simulink model "IM2_IndirectVector"  (R2022a)
settings: Solver=ode45  StartTime=0.0  StopTime=2  MaxStep=1e-5  RelTol=1e-3
values from neighbouring files (symbols this model uses):
  Vdc = 300    [IM2_Vector.m]    (also in Induction_motor_parameter.m)
undefined symbols (not defined in the file or in its folder): DCMotor, DiscIntNeverNeededParam, IM, INV1, INV2
libraries: simulink x3
settings Model: Creator=jun  LastModifiedBy=jun
settings DebuggingCC: UnconnectedInputMsg=warning  UnconnectedOutputMsg=warning  UnconnectedLineMsg=warning
settings RTWCC: DLArmComputeVersion=19.05

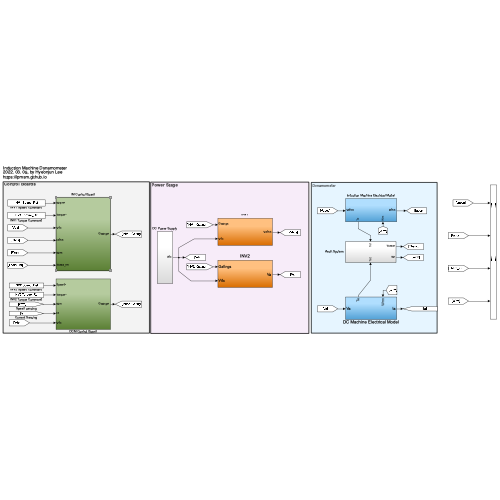
[thumbnail: Simulink's stored preview of the top-level diagram]
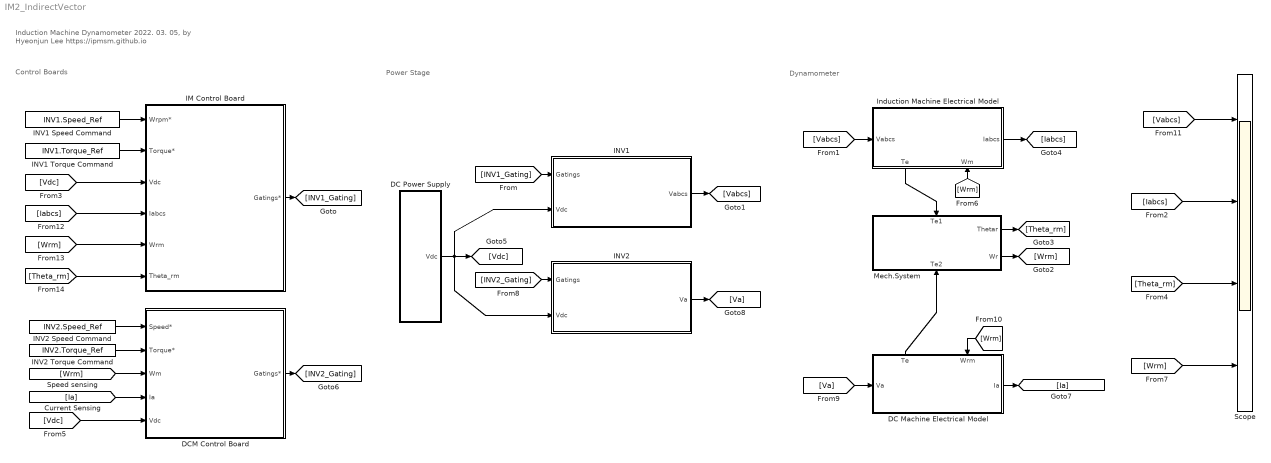
== system IM2_IndirectVector ==
  note: Induction Machine Dynamometer
      | 2022. 03. 05, by Hyeonjun Lee
      | https://ipmsm.github.io
  note: Dynamometer
  note: Power Stage
  note: Control Boards
  DC Machine Electrical Model : Subsystem
      settings: PortSchema="{\"entries\":[{\"content\":{\"sides\":[{\"content\":{\"connectorIds\":[\"In1\"]},\"type\":\"ConnectorPlacement.EquallySpacedRectSide\",\"uuid\":\"4074897e-6920-4f33-b302-64d86120b7df\"},{\"content\":{\"connectorIds\":[\"Out1\"],\"side\":\"RIGHT\"},\"type\":\"ConnectorPlacement.EquallySpacedRectSide\",\"uuid\":\"671615ca-e362-48c9-a030-03d33faae874\"},{\"content\":{\"connectorIds\":[\"Out2\",\"In2\"],\"side\":\"TOP\"},\"type\":\"ConnectorPlacement.EquallySpacedRectSide\",\"uuid\":\"d587e8fb-b462-47db-b9f9-66f25c83a3fe\"},{\"content\":{\"connectorIds\":[],\"side\":\"BOTTOM\"},\"type\":\"ConnectorPlacement.EquallySpacedRectSide\",\"uuid\":\"9be21003-cb0d-41fd-b790-e70774da76cb\"}]},\"type\":\"ConnectorPlacement.EquallySpacedConnector\",\"uuid\":\"22d4a5b5-b610-40ac-ac45-102e1f1adc00\"}],\"packageUris\":[\"http://schema.mathworks.com/mf0/Connector/R2020b\"],\"version\":\"1.0\"}"
  DC Power Supply : Subsystem
  DCM Control Board : Subsystem
  IM Control Board : Subsystem
  INV1 : Subsystem
  INV1 Speed Command : Constant  Value=INV1.Speed_Ref
  INV1 Torque Command : Constant  Value=INV1.Torque_Ref
  INV2 : Subsystem
  INV2 Speed Command : Constant  Value=INV2.Speed_Ref
  INV2 Torque Command : Constant  Value=INV2.Torque_Ref
  Induction Machine Electrical Model : Subsystem
      settings: PortSchema="{\"entries\":[{\"content\":{\"sides\":[{\"content\":{\"connectorIds\":[\"In1\"]},\"type\":\"ConnectorPlacement.EquallySpacedRectSide\",\"uuid\":\"2d22a4ac-8ce0-4f43-8306-e5d06343ee91\"},{\"content\":{\"connectorIds\":[\"Out1\"],\"side\":\"RIGHT\"},\"type\":\"ConnectorPlacement.EquallySpacedRectSide\",\"uuid\":\"eaa0b2e3-b8a8-4ec2-a419-1e6d0efc2421\"},{\"content\":{\"connectorIds\":[],\"side\":\"TOP\"},\"type\":\"ConnectorPlacement.EquallySpacedRectSide\",\"uuid\":\"755c15fe-a709-466a-9725-b33f4e12c3a1\"},{\"content\":{\"connectorIds\":[\"Out2\",\"In2\"],\"side\":\"BOTTOM\"},\"type\":\"ConnectorPlacement.EquallySpacedRectSide\",\"uuid\":\"8ffd0ea7-af21-4bb6-bd52-5cb3d0234bc0\"}]},\"type\":\"ConnectorPlacement.EquallySpacedConnector\",\"uuid\":\"5b0edaea-9abe-4353-a27d-04fae1d4b959\"}],\"packageUris\":[\"http://schema.mathworks.com/mf0/Connector/R2020b\"],\"version\":\"1.0\"}"
  Mech.System : Subsystem
      settings: PortSchema="{\"entries\":[{\"content\":{\"sides\":[{\"content\":{\"connectorIds\":[]},\"type\":\"ConnectorPlacement.EquallySpacedRectSide\",\"uuid\":\"7816393c-e6ef-44df-b641-25156ded1cdc\"},{\"content\":{\"connectorIds\":[\"Out1\",\"Out2\"],\"side\":\"RIGHT\"},\"type\":\"ConnectorPlacement.EquallySpacedRectSide\",\"uuid\":\"df3d9513-253d-4c97-8efd-af2438fb286e\"},{\"content\":{\"connectorIds\":[\"In1\"],\"side\":\"TOP\"},\"type\":\"ConnectorPlacement.EquallySpacedRectSide\",\"uuid\":\"65b6b526-a008-40f6-a42d-b2e1dc0c5f24\"},{\"content\":{\"connectorIds\":[\"In2\"],\"side\":\"BOTTOM\"},\"type\":\"ConnectorPlacement.EquallySpacedRectSide\",\"uuid\":\"f448aff5-19c1-43a0-84ba-52356c379f88\"}]},\"type\":\"ConnectorPlacement.EquallySpacedConnector\",\"uuid\":\"afd6e091-39ce-476c-80f4-568492feeb85\"}],\"packageUris\":[\"http://schema.mathworks.com/mf0/Connector/R2020b\"],\"version\":\"1.0\"}"
  Scope : Scope  NumInputPorts=4
  wires:
  INV1 Speed Command/1 -> IM Control Board/1(Wrpm*)
  IM Control Board/1(Gatings*) -> [INV1_Gating]
  [INV1_Gating] -> INV1/1(Gatings)
  [Vabcs] -> Induction Machine Electrical Model/1(Vabcs)
  Induction Machine Electrical Model/2(Te) -> Mech.System/1(Te1)
  Induction Machine Electrical Model/1(Iabcs) -> [Iabcs]
  [Vdc] -> IM Control Board/3(Vdc)
  INV2 Speed Command/1 -> DCM Control Board/1(Speed*)
  [Wrm] -> DCM Control Board/3(Wm)
  [Ia] -> DCM Control Board/4(Ia)
  DCM Control Board/1(Gatings*) -> [INV2_Gating]
  INV2 Torque Command/1 -> DCM Control Board/2(Torque*)
  [Vdc] -> DCM Control Board/5(Vdc)
  [INV2_Gating] -> INV2/1(Gatings)
  DC Machine Electrical Model/2(Te) -> Mech.System/2(Te2)
  Mech.System/1(Thetar) -> [Theta_rm]
  [Wrm] -> Induction Machine Electrical Model/2(Wm)
  Mech.System/2(Wr) -> [Wrm]
  [Va] -> DC Machine Electrical Model/1(Va)
  INV2/1(Va) -> [Va]
  DC Power Supply/1(Vdc) -> INV1/2(Vdc), [Vdc], INV2/2(Vdc)
  [Iabcs] -> Scope/2
  [Theta_rm] -> Scope/3
  [Wrm] -> Scope/4
  INV1/1(Vabcs) -> [Vabcs]
  [Wrm] -> DC Machine Electrical Model/2(Wrm)
  [Vabcs] -> Scope/1
  DC Machine Electrical Model/1(Ia) -> [Ia]
  INV1 Torque Command/1 -> IM Control Board/2(Torque*)
  [Iabcs] -> IM Control Board/4(Iabcs)
  [Wrm] -> IM Control Board/5(Wrm)
  [Theta_rm] -> IM Control Board/6(Theta_rm)

== system IM2_IndirectVector/DC Machine Electrical Model ==
  note: DC Machine Mech Model
  note: DC Machine Electrical Model
  Va : Inport
  Wrm : Inport  Port=2
  1/La2 : Gain  Gain=DCMotor.K  SaturateOnIntegerOverflow=on  OutDataTypeStr=Inherit: Same as input  ParamDataTypeStr=Inherit: Same as input
  Gain2 : Gain  Gain=1/DCMotor.La
  Gain3 : Gain  Gain=DCMotor.Ra
  Gain4 : Gain  Gain=DCMotor.K
  Integrator1 : Integrator
  Sum : Sum  Inputs=+--  SaturateOnIntegerOverflow=on
  Ia : Outport
  Te : Outport  Port=2  VectorParamsAs1DForOutWhenUnconnected=off
  wires:
  1/La2/1 -> Sum/2
  Integrator1/1 -> Gain4/1, Ia/1, Gain3/1
  Sum/1 -> Gain2/1
  Gain4/1 -> [Te], Te/1
  Va/1 -> Sum/1
  Gain2/1 -> Integrator1/1
  Gain3/1 -> Sum/3
  Wrm/1 -> 1/La2/1

== system IM2_IndirectVector/DC Power Supply ==
  Constant : Constant  Value=Vdc
  Vdc : Outport
  wires:
  Constant/1 -> Vdc/1

== system IM2_IndirectVector/DCM Control Board ==
  Speed* : Inport
  Torque* : Inport  Port=2
  Wm : Inport  Port=3
  Ia : Inport  Port=4
  Vdc : Inport  Port=5
  Control Programs : Subsystem
  Fsw : DiscretePulseGenerator  PulseType=Time based  Period=1/INV2.SwitchingFrequency  PulseWidth=50
  Gain : Gain  Gain=-1
  PWM Module : Subsystem
  Gatings* : Outport
  wires:
  PWM Module/1(Gating) -> Gatings*/1
  Speed*/1 -> Control Programs/1(Speed*)
  Torque*/1 -> Control Programs/2(Torque*)
  Wm/1 -> Gain/1
  Ia/1 -> Control Programs/4(Ia)
  Fsw/1 -> Control Programs/Trigger
  Control Programs/1(Counter) -> PWM Module/1(Counter)
  Vdc/1 -> Control Programs/5(Vdc)
  Gain/1 -> Control Programs/3(Wm)

== system IM2_IndirectVector/IM Control Board ==
  Wrpm* : Inport
  Torque* : Inport  Port=2
  Vdc : Inport  Port=3
  Iabcs : Inport  Port=4
  Wrm : Inport  Port=5
  Theta_rm : Inport  Port=6
  Control Programs : Subsystem
  Fsw : DiscretePulseGenerator  PulseType=Time based  Period=INV1.Tsw  PulseWidth=50
  PWM Module : Subsystem
  Gatings* : Outport
  wires:
  Wrpm*/1 -> Control Programs/1(Wrpm*)
  Vdc/1 -> Control Programs/5(Vdc)
  Control Programs/1(Counter) -> PWM Module/1(Counter)
  PWM Module/1(Gatings) -> Gatings*/1
  Fsw/1 -> Control Programs/Trigger
  Torque*/1 -> Control Programs/2(Te*)
  Iabcs/1 -> Control Programs/3(Iabcs)
  Wrm/1 -> Control Programs/4(Wrm)
  Theta_rm/1 -> Control Programs/6(Theta_rm)

== system IM2_IndirectVector/INV1 ==
  Gatings : Inport
  Vdc : Inport  Port=2
  Product : Product
  Vabcs : Outport
  wires:
  Gatings/1 -> Product/1
  Vdc/1 -> Product/2
  Product/1 -> Vabcs/1

== system IM2_IndirectVector/INV2 ==
  Gatings : Inport
  Vdc : Inport  Port=2
  Product : Product
  Va : Outport  InitialOutput=0  VectorParamsAs1DForOutWhenUnconnected=off
  wires:
  Vdc/1 -> Product/2
  Product/1 -> Va/1
  Gatings/1 -> Product/1

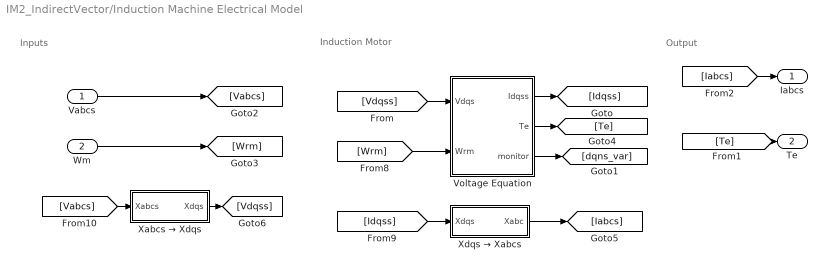
== system IM2_IndirectVector/Induction Machine Electrical Model ==
  note: Output
  note: Inputs
  note: Induction Motor
  Vabcs : Inport
  Wm : Inport  Port=2
  Voltage Equation : Subsystem
  Xabcs → Xdqs : Subsystem
  Xdqs → Xabcs : Subsystem
  Iabcs : Outport
  Te : Outport  Port=2
  wires:
  Voltage Equation/2(Te) -> [Te]
  Voltage Equation/3(monitor) -> [dqns_var]
  Vabcs/1 -> [Vabcs]
  [Vdqss] -> Voltage Equation/1(Vdqs)
  Voltage Equation/1(Idqss) -> [Idqss]
  Wm/1 -> [Wrm]
  [Wrm] -> Voltage Equation/2(Wrm)
  [Idqss] -> Xdqs → Xabcs/1(Xdqs)
  Xdqs → Xabcs/1(Xabc) -> [Iabcs]
  [Vabcs] -> Xabcs → Xdqs/1(Xabcs)
  Xabcs → Xdqs/1(Xdqs) -> [Vdqss]
  [Te] -> Te/1
  [Iabcs] -> Iabcs/1

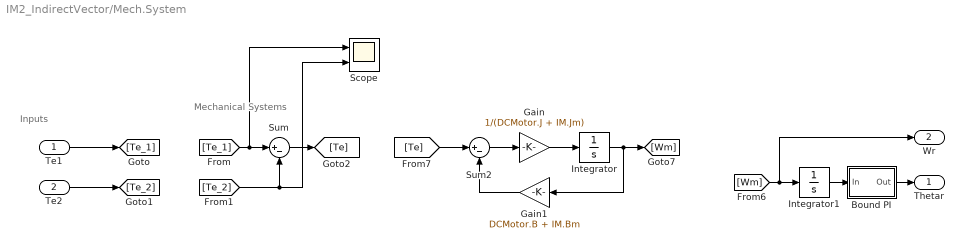
== system IM2_IndirectVector/Mech.System ==
  note: Mechanical Systems
  note: Inputs
  Te1 : Inport
  Te2 : Inport  Port=2
  Bound PI : Subsystem
  Gain : Gain  Gain=1/(DCMotor.J + IM.Jm)
  Gain1 : Gain  Gain=DCMotor.B + IM.Bm
  Integrator : Integrator
  Integrator1 : Integrator
  Scope : Scope  NumInputPorts=2
  Sum : Sum  Inputs=|+-
  Sum2 : Sum  Inputs=|+-
  Thetar : Outport  VectorParamsAs1DForOutWhenUnconnected=off
  Wr : Outport  Port=2
  wires:
  Sum2/1 -> Gain/1
  Gain1/1 -> Sum2/2
  Gain/1 -> Integrator/1
  Integrator/1 -> Gain1/1, [Wm]
  Te1/1 -> [Te_1]
  Te2/1 -> [Te_2]
  [Te_1] -> Scope/1, Sum/1
  [Te_2] -> Scope/2, Sum/2
  Sum/1 -> [Te]
  [Te] -> Sum2/1
  Bound PI/1(Out) -> Thetar/1
  Integrator1/1 -> Bound PI/1(In)
  [Wm] -> Wr/1, Integrator1/1

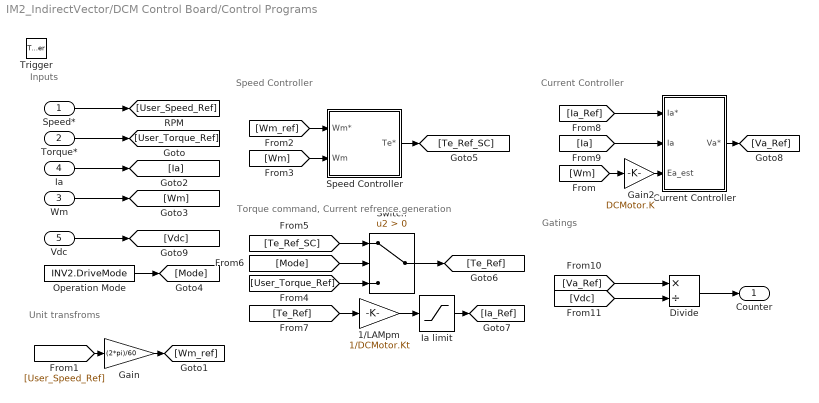
== system IM2_IndirectVector/DCM Control Board/Control Programs ==
  note: Speed Controller
  note: Unit transfroms
  note: Inputs
  note: Current Controller
  note: Gatings
  note: Torque command, Current refrence generation
  Speed* : Inport
  Torque* : Inport  Port=2
  Wm : Inport  Port=3
  Ia : Inport  Port=4
  Vdc : Inport  Port=5
  Trigger : TriggerPort  VariantControl=(inherit)  PortDimensions=1
  1/LAMpm : Gain  Gain=1/DCMotor.Kt  SaturateOnIntegerOverflow=on  OutDataTypeStr=Inherit: Same as input  ParamDataTypeStr=Inherit: Same as input
  Current Controller : Subsystem
  Divide : Product  Inputs=*/
  Gain : Gain  Gain=(2*pi)/60
  Gain2 : Gain  Gain=DCMotor.K
  Ia limit : Saturate  UpperLimit=DCMotor.Ia_limit  LowerLimit=-DCMotor.Ia_limit
  Operation Mode : Constant  Value=INV2.DriveMode
  Speed Controller : Subsystem
  Switch : Switch  Criteria=u2 > Threshold  SaturateOnIntegerOverflow=off  InputSameDT=off
  Counter : Outport
  wires:
  Speed*/1 -> [User_Speed_Ref]
  Gain/1 -> [Wm_ref]
  Gain2/1 -> Current Controller/3(Ea_est)
  Torque*/1 -> [User_Torque_Ref]
  [Te_Ref] -> 1/LAMpm/1
  Current Controller/1(Va*) -> [Va_Ref]
  Speed Controller/1(Te*) -> [Te_Ref_SC]
  Ia/1 -> [Ia]
  [Ia_Ref] -> Current Controller/1(Ia*)
  Switch/1 -> [Te_Ref]
  [Ia] -> Current Controller/2(Ia)
  [Mode] -> Switch/2
  Ia limit/1 -> [Ia_Ref]
  Operation Mode/1 -> [Mode]
  [User_Torque_Ref] -> Switch/3
  [Wm] -> Gain2/1
  1/LAMpm/1 -> Ia limit/1
  [User_Speed_Ref] -> Gain/1
  [Te_Ref_SC] -> Switch/1
  [Wm] -> Speed Controller/2(Wm)
  [Wm_ref] -> Speed Controller/1(Wm*)
  Wm/1 -> [Wm]
  Vdc/1 -> [Vdc]
  [Va_Ref] -> Divide/1
  Divide/1 -> Counter/1
  [Vdc] -> Divide/2

== system IM2_IndirectVector/DCM Control Board/PWM Module ==
  Counter : Inport
  1/3 : Gain  Gain=-1  SaturateOnIntegerOverflow=on  OutDataTypeStr=Inherit: Same as input  ParamDataTypeStr=Inherit: Same as input
  Carrier wave : simulink/Sources/Repeating Sequence  rep_seq_t="[0  1/2/INV2.SwitchingFrequency  1/INV2.SwitchingFrequency]"  rep_seq_y=[-1 1 -1]
  Relational Operator : RelationalOperator
  Relational Operator1 : RelationalOperator
  Sum2 : Sum  Inputs=+-  SaturateOnIntegerOverflow=on
  Gating : Outport
  wires:
  Counter/1 -> 1/3/1, Relational Operator/1
  Relational Operator/1 -> Sum2/1
  Sum2/1 -> Gating/1
  Carrier wave/1 -> Relational Operator1/2, Relational Operator/2
  Relational Operator1/1 -> Sum2/2
  1/3/1 -> Relational Operator1/1

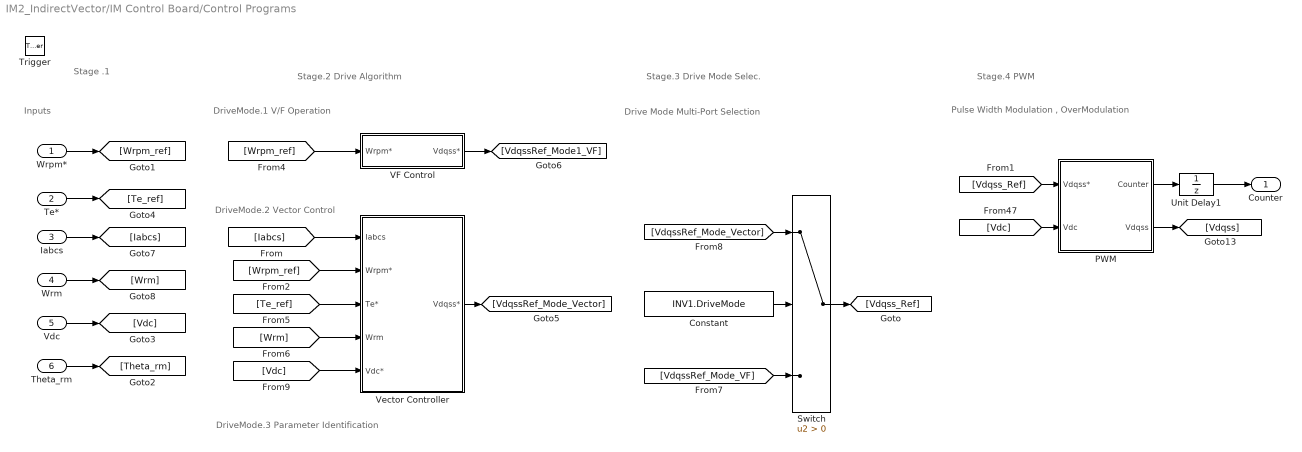
== system IM2_IndirectVector/IM Control Board/Control Programs ==
  note: DriveMode.3 Parameter Identification
  note: Pulse Width Modulation , OverModulation
  note: Stage .1
  note: DriveMode.2 Vector Control
  note: Drive Mode Multi-Port Selection
  note: DriveMode.1 V/F Operation
  note: Inputs
  note: Stage.2 Drive Algorithm
  note: Stage.3 Drive Mode Selec.
  note: Stage.4 PWM
  Wrpm* : Inport
  Te* : Inport  Port=2
  Iabcs : Inport  Port=3
  Wrm : Inport  Port=4
  Vdc : Inport  Port=5
  Theta_rm : Inport  Port=6
  Trigger : TriggerPort  VariantControl=(inherit)  PortDimensions=1
  Constant : Constant  Value=INV1.DriveMode
  PWM : Subsystem
  Switch : Switch  Criteria=u2 > Threshold  SaturateOnIntegerOverflow=off  InputSameDT=off
  Unit Delay1 : UnitDelay  SampleTime=-1  HasFrameUpgradeWarning=on
  VF Control : Subsystem
  Vector Controller : Subsystem
  Counter : Outport
  wires:
  Vdc/1 -> [Vdc]
  VF Control/1(Vdqss*) -> [VdqssRef_Mode1_VF]
  PWM/1(Counter) -> Unit Delay1/1
  Unit Delay1/1 -> Counter/1
  [Vdqss_Ref] -> PWM/1(Vdqss*)
  PWM/2(Vdqss) -> [Vdqss]
  Wrpm*/1 -> [Wrpm_ref]
  [Vdc] -> PWM/2(Vdc)
  [Wrpm_ref] -> VF Control/1(Wrpm*)
  Te*/1 -> [Te_ref]
  Iabcs/1 -> [Iabcs]
  Wrm/1 -> [Wrm]
  [Iabcs] -> Vector Controller/1(Iabcs)
  [Wrpm_ref] -> Vector Controller/2(Wrpm*)
  [Te_ref] -> Vector Controller/3(Te*)
  [Wrm] -> Vector Controller/4(Wrm)
  [Vdc] -> Vector Controller/5(Vdc*)
  Theta_rm/1 -> [Theta_rm]
  [VdqssRef_Mode_VF] -> Switch/3
  [VdqssRef_Mode_Vector] -> Switch/1
  Switch/1 -> [Vdqss_Ref]
  Vector Controller/1(Vdqss*) -> [VdqssRef_Mode_Vector]
  Constant/1 -> Switch/2

== system IM2_IndirectVector/IM Control Board/PWM Module ==
  Counter : Inport
  Add3 : Sum  Inputs=+-
  Relay3 : Relay  OnSwitchValue=10*eps  OffSwitchValue=-10*eps  OutDataTypeStr=double
  Repeating Sequence1 : simulink/Sources/Repeating Sequence  rep_seq_t=[0 INV1.Tsw/2 INV1.Tsw]  rep_seq_y=[0 1 0]
  Gatings : Outport
  wires:
  Add3/1 -> Relay3/1
  Relay3/1 -> Gatings/1
  Repeating Sequence1/1 -> Add3/2
  Counter/1 -> Add3/1

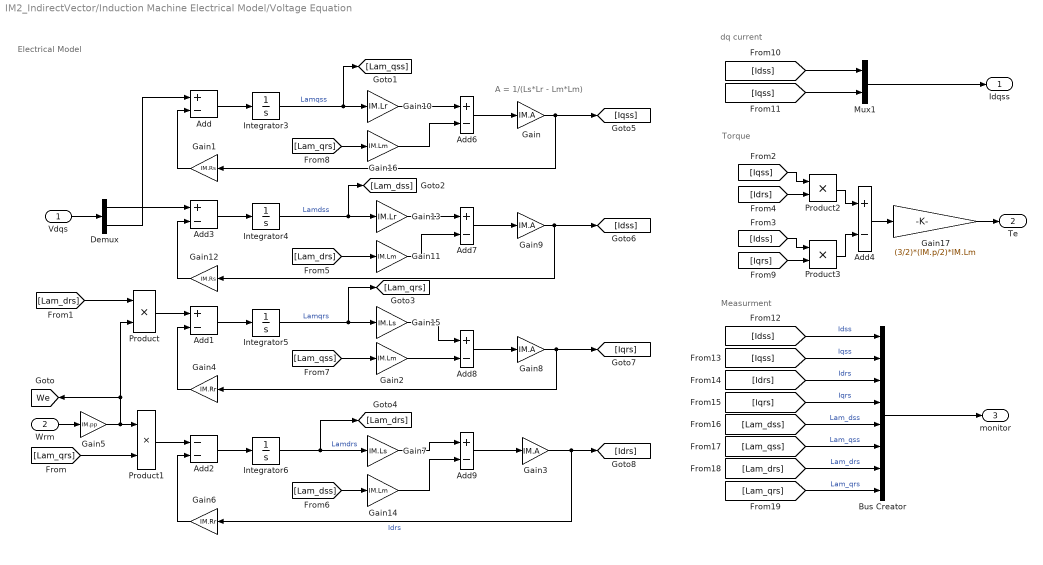
== system IM2_IndirectVector/Induction Machine Electrical Model/Voltage Equation ==
  note: Measurment
  note: dq current
  note: Torque
  note: Electrical Model
  note: A = 1/(Ls*Lr - Lm*Lm)
  Vdqs : Inport
  Wrm : Inport  Port=2
  Add{,1,3..4,6..9} (8 alike) : Sum  Inputs=+-
  Add2 : Sum  Inputs=--
  Bus Creator : BusCreator  Inputs=8
  Demux : Demux  Outputs=2
  Gain{,3,8..9} (4 alike) : Gain  Gain=IM.A
  Gain1 : Gain  Gain=IM.Rs
  Gain10 : Gain  Gain=IM.Lr
  Gain{2,11,14,16} (4 alike) : Gain  Gain=IM.Lm
  Gain12 : Gain  Gain=IM.Rs
  Gain13 : Gain  Gain=IM.Lr
  Gain15 : Gain  Gain=IM.Ls
  Gain17 : Gain  Gain=(3/2)*(IM.p/2)*IM.Lm
  Gain4 : Gain  Gain=IM.Rr
  Gain5 : Gain  Gain=IM.pp
  Gain6 : Gain  Gain=IM.Rr
  Gain7 : Gain  Gain=IM.Ls
  Integrator{3..6} (4 alike) : Integrator
  Mux1 : Mux  Inputs=2
  Product{,1..3} (4 alike) : Product
  Idqss : Outport  VectorParamsAs1DForOutWhenUnconnected=off
  Te : Outport  Port=2  VectorParamsAs1DForOutWhenUnconnected=off
  monitor : Outport  Port=3  VectorParamsAs1DForOutWhenUnconnected=off
  tag scope: We=global
  wires:
  Gain/1 -> Gain1/1, [Iqss]
  Wrm/1 -> Gain5/1
  Integrator3/1 -> [Lam_qss], Gain10/1  "Lamqss"
  Integrator4/1 -> [Lam_dss], Gain13/1  "Lamdss"
  Integrator5/1 -> [Lam_qrs], Gain15/1  "Lamqrs"
  Integrator6/1 -> [Lam_drs], Gain7/1  "Lamdrs"
  Gain9/1 -> Gain12/1, [Idss]
  Gain8/1 -> [Iqrs], Gain4/1
  Gain3/1 -> [Idrs], Gain6/1  "Idrs"
  Add6/1 -> Gain/1
  Add7/1 -> Gain9/1
  Add8/1 -> Gain8/1
  Add9/1 -> Gain3/1
  Gain10/1 -> Add6/1
  Add/1 -> Integrator3/1
  Gain1/1 -> Add/2
  Add1/1 -> Integrator5/1
  Gain4/1 -> Add1/2
  Product/1 -> Add1/1
  Gain5/1 -> Product/2, [We], Product1/1
  Add2/1 -> Integrator6/1
  Gain6/1 -> Add2/2
  Gain7/1 -> Add9/1
  Add3/1 -> Integrator4/1
  Gain12/1 -> Add3/2
  Gain13/1 -> Add7/1
  Product1/1 -> Add2/1
  Demux/2 -> Add/1
  Gain17/1 -> Te/1
  Add4/1 -> Gain17/1
  Product2/1 -> Add4/1
  Product3/1 -> Add4/2
  [Lam_qrs] -> Product1/2
  [Lam_drs] -> Product/1
  [Iqss] -> Product2/1
  [Idss] -> Product3/1
  [Iqrs] -> Product3/2
  Gain11/1 -> Add7/2
  [Lam_drs] -> Gain11/1
  [Lam_dss] -> Gain14/1
  Gain16/1 -> Add6/2
  [Lam_qss] -> Gain2/1
  Gain15/1 -> Add8/1
  Gain2/1 -> Add8/2
  [Lam_qrs] -> Gain16/1
  [Idrs] -> Product2/2
  Gain14/1 -> Add9/2
  [Idss] -> Mux1/1
  [Iqss] -> Mux1/2
  Mux1/1 -> Idqss/1
  [Idss] -> Bus Creator/1  "Idss"
  [Iqss] -> Bus Creator/2  "Iqss"
  [Idrs] -> Bus Creator/3  "Idrs"
  [Iqrs] -> Bus Creator/4  "Iqrs"
  [Lam_dss] -> Bus Creator/5  "Lam_dss"
  [Lam_qss] -> Bus Creator/6  "Lam_qss"
  [Lam_drs] -> Bus Creator/7  "Lam_drs"
  [Lam_qrs] -> Bus Creator/8  "Lam_qrs"
  Bus Creator/1 -> monitor/1
  Vdqs/1 -> Demux/1
  Demux/1 -> Add3/1

== system IM2_IndirectVector/Induction Machine Electrical Model/Xabcs → Xdqs ==
  Xabcs : Inport
  Add : Sum  Inputs=+--
  Add1 : Sum  Inputs=+-
  Demux : Demux  Outputs=3
  Gain : Gain  Gain=2
  Gain1 : Gain  Gain=1/3
  Gain2 : Gain  Gain=1/sqrt(3)
  Mux : Mux  Inputs=2
  Xdqs : Outport  VectorParamsAs1DForOutWhenUnconnected=off
  wires:
  Demux/1 -> Gain/1
  Gain/1 -> Add/1
  Demux/2 -> Add1/1, Add/2
  Demux/3 -> Add1/2, Add/3
  Add/1 -> Gain1/1
  Gain1/1 -> Mux/1
  Gain2/1 -> Mux/2
  Add1/1 -> Gain2/1
  Mux/1 -> Xdqs/1
  Xabcs/1 -> Demux/1

== system IM2_IndirectVector/Induction Machine Electrical Model/Xdqs → Xabcs ==
  Xdqs : Inport
  Add : Sum  Inputs=-+
  Add1 : Sum  Inputs=--
  Demux : Demux  Outputs=2
  Gain : Gain  Gain=1/2
  Gain1 : Gain  Gain=sqrt(3)/2
  Mux : Mux  Inputs=3
  Xabc : Outport  VectorParamsAs1DForOutWhenUnconnected=off
  wires:
  Demux/1 -> Mux/1, Gain/1
  Add/1 -> Mux/2
  Add1/1 -> Mux/3
  Demux/2 -> Gain1/1
  Gain1/1 -> Add1/2, Add/2
  Gain/1 -> Add1/1, Add/1
  Mux/1 -> Xabc/1
  Xdqs/1 -> Demux/1

== system IM2_IndirectVector/Mech.System/Bound PI ==
  In : Inport
  Fcn1 : Fcn  Expr=1/(2*pi)*u+0.5
  Fcn2 : Fcn  Expr=u-floor(u)
  Fcn3 : Fcn  Expr=2*pi*(u-0.5)
  Out : Outport
  wires:
  Fcn1/1 -> Fcn2/1
  Fcn2/1 -> Fcn3/1
  In/1 -> Fcn1/1
  Fcn3/1 -> Out/1

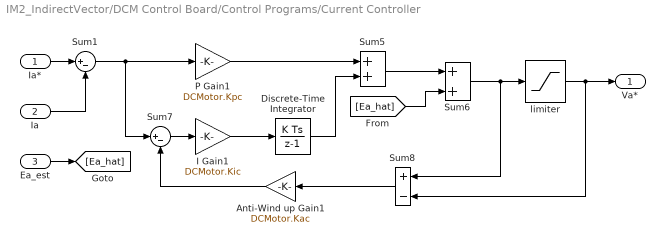
== system IM2_IndirectVector/DCM Control Board/Control Programs/Current Controller ==
  Ia* : Inport
  Ia : Inport  Port=2
  Ea_est : Inport  Port=3
  Anti-Wind up Gain1 : Gain  Gain=DCMotor.Kac  SaturateOnIntegerOverflow=on  OutDataTypeStr=Inherit: Same as input  ParamDataTypeStr=Inherit: Same as input
  Discrete-Time Integrator : DiscreteIntegrator  SampleTime=-1  ICPrevOutput=DiscIntNeverNeededParam  ICPrevScaledInput=DiscIntNeverNeededParam
  I Gain1 : Gain  Gain=DCMotor.Kic  SaturateOnIntegerOverflow=on  OutDataTypeStr=Inherit: Same as input  ParamDataTypeStr=Inherit: Same as input
  P Gain1 : Gain  Gain=DCMotor.Kpc  SaturateOnIntegerOverflow=on  OutDataTypeStr=Inherit: Same as input  ParamDataTypeStr=Inherit: Same as input
  Sum1 : Sum  Inputs=|+-  SaturateOnIntegerOverflow=on
  Sum5 : Sum  SaturateOnIntegerOverflow=on
  Sum6 : Sum  SaturateOnIntegerOverflow=on
  Sum7 : Sum  Inputs=|+-  SaturateOnIntegerOverflow=on
  Sum8 : Sum  Inputs=+-  SaturateOnIntegerOverflow=on
  limiter : Saturate  UpperLimit=DCMotor.Va_rated  LowerLimit=-DCMotor.Va_rated
  Va* : Outport  VectorParamsAs1DForOutWhenUnconnected=off
  wires:
  limiter/1 -> Va*/1, Sum8/2
  Sum8/1 -> Anti-Wind up Gain1/1
  Anti-Wind up Gain1/1 -> Sum7/2
  Sum7/1 -> I Gain1/1
  Sum1/1 -> Sum7/1, P Gain1/1
  P Gain1/1 -> Sum5/1
  Discrete-Time Integrator/1 -> Sum5/2
  Sum5/1 -> Sum6/1
  Sum6/1 -> limiter/1, Sum8/1
  I Gain1/1 -> Discrete-Time Integrator/1
  Ia*/1 -> Sum1/1
  [Ea_hat] -> Sum6/2
  Ia/1 -> Sum1/2
  Ea_est/1 -> [Ea_hat]

== system IM2_IndirectVector/DCM Control Board/Control Programs/Speed Controller ==
  note: Te*
  Wm* : Inport
  Wm : Inport  Port=2
  Discrete-Time Integrator : DiscreteIntegrator  SampleTime=-1  ICPrevOutput=DiscIntNeverNeededParam  ICPrevScaledInput=DiscIntNeverNeededParam
  Ksa : Gain  Gain=DCMotor.Ksa  SaturateOnIntegerOverflow=on  OutDataTypeStr=Inherit: Same as input  ParamDataTypeStr=Inherit: Same as input
  Ksi : Gain  Gain=DCMotor.Ksi  SaturateOnIntegerOverflow=on  OutDataTypeStr=Inherit: Same as input  ParamDataTypeStr=Inherit: Same as input
  Ksp : Gain  Gain=DCMotor.Ksp  SaturateOnIntegerOverflow=on  OutDataTypeStr=Inherit: Same as input  ParamDataTypeStr=Inherit: Same as input
  Sum : Sum  Inputs=|+-  SaturateOnIntegerOverflow=on
  Sum2 : Sum  Inputs=|+-  SaturateOnIntegerOverflow=on
  Sum3 : Sum  Inputs=++|  SaturateOnIntegerOverflow=on
  Sum4 : Sum  Inputs=+-  SaturateOnIntegerOverflow=on
  Te-limiter : Saturate  UpperLimit=DCMotor.Te_limit  LowerLimit=-DCMotor.Te_limit
  Te* : Outport  VectorParamsAs1DForOutWhenUnconnected=off
  wires:
  Ksa/1 -> Sum2/2
  Sum2/1 -> Ksi/1
  Sum4/1 -> Ksa/1
  Sum/1 -> Sum2/1, Ksp/1
  Ksi/1 -> Discrete-Time Integrator/1
  Ksp/1 -> Sum3/1
  Discrete-Time Integrator/1 -> Sum3/2
  Sum3/1 -> Sum4/1, Te-limiter/1
  Wm/1 -> Sum/2
  Te-limiter/1 -> Te*/1, Sum4/2
  Wm*/1 -> Sum/1

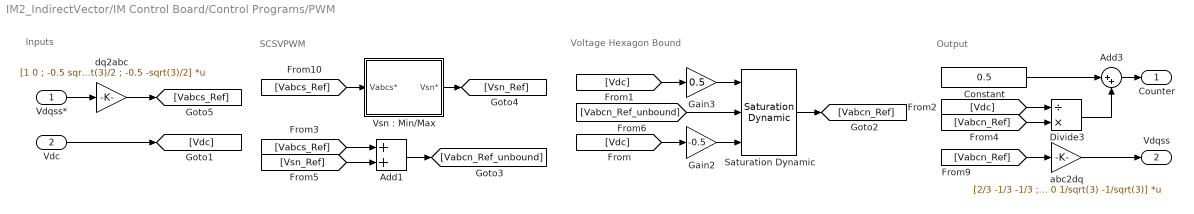
== system IM2_IndirectVector/IM Control Board/Control Programs/PWM ==
  note: Output
  note: Voltage Hexagon Bound
  note: SCSVPWM
  note: Inputs
  Vdqss* : Inport
  Vdc : Inport  Port=2
  Add1 : Sum
  Add3 : Sum  Inputs=|++
  Constant : Constant  Value=0.5
  Divide3 : Product  Inputs=/*
  Gain2 : Gain  Gain=-0.5
  Gain3 : Gain  Gain=0.5
  Saturation Dynamic : simulink/Discontinuities/Saturation Dynamic  OutMin=[]  OutMax=[]  OutDataTypeStr=Inherit: Same as second input  OutDataType=fixdt(1, 16)  OutScaling=2^-10  DoSatur=off
  "Vsn : Min/Max" : Subsystem
  abc2dq : Gain  Gain=[2/3 -1/3 -1/3 ; 0 1/sqrt(3) -1/sqrt(3)]  Multiplication=Matrix(K*u)  SaturateOnIntegerOverflow=on  OutDataTypeStr=Inherit: Same as input  ParamDataTypeStr=Inherit: Same as input
  dq2abc : Gain  Gain=[1 0 ; -0.5 sqrt(3)/2 ; -0.5 -sqrt(3)/2]  Multiplication=Matrix(K*u)
  Counter : Outport
  Vdqss : Outport  Port=2
  wires:
  Vdqss*/1 -> dq2abc/1
  dq2abc/1 -> [Vabcs_Ref]
  Gain2/1 -> Saturation Dynamic/3
  Vdc/1 -> [Vdc]
  Saturation Dynamic/1 -> [Vabcn_Ref]
  abc2dq/1 -> Vdqss/1
  [Vabcn_Ref] -> abc2dq/1
  [Vabcs_Ref] -> "Vsn : Min/Max"/1(Vabcs*)
  "Vsn : Min/Max"/1(Vsn*) -> [Vsn_Ref]
  Divide3/1 -> Add3/2
  [Vabcn_Ref] -> Divide3/2
  Constant/1 -> Add3/1
  Add3/1 -> Counter/1
  [Vdc] -> Divide3/1
  [Vabcs_Ref] -> Add1/1
  [Vsn_Ref] -> Add1/2
  Add1/1 -> [Vabcn_Ref_unbound]
  [Vdc] -> Gain2/1
  Gain3/1 -> Saturation Dynamic/1
  [Vdc] -> Gain3/1
  [Vabcn_Ref_unbound] -> Saturation Dynamic/2

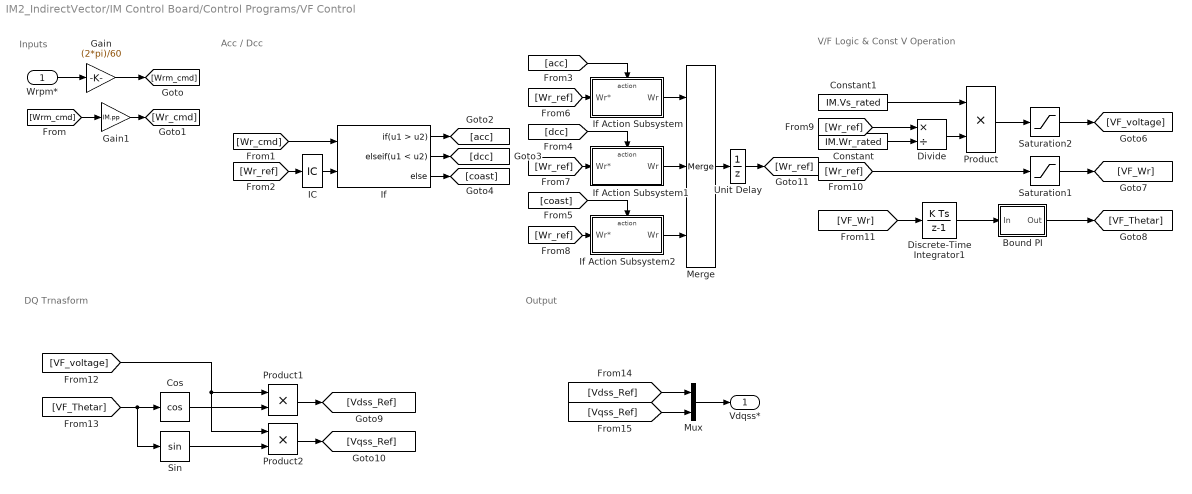
== system IM2_IndirectVector/IM Control Board/Control Programs/VF Control ==
  note: Output
  note: DQ Trnasform
  note: V/F Logic & Const V Operation
  note: Acc / Dcc
  note: Inputs
  Wrpm* : Inport
  Bound PI : Subsystem
  Constant : Constant  Value=IM.Wr_rated
  Constant1 : Constant  Value=IM.Vs_rated
  Cos : Trigonometry  Operator=cos
  Discrete-Time Integrator1 : DiscreteIntegrator  SampleTime=-1  ICPrevOutput=DiscIntNeverNeededParam  ICPrevScaledInput=DiscIntNeverNeededParam
  Divide : Product  Inputs=*/
  Gain : Gain  Gain=(2*pi)/60
  Gain1 : Gain  Gain=IM.pp
  IC : InitialCondition  Value=0
  If : If  NumInputs=2  IfExpression=u1 > u2  ElseIfExpressions=u1 < u2
  If Action Subsystem : Subsystem  TreatAsAtomicUnit=on
  If Action Subsystem1 : Subsystem  TreatAsAtomicUnit=on
  If Action Subsystem2 : Subsystem  TreatAsAtomicUnit=on
  Merge : Merge  Inputs=3  InitialOutput=[1]
  Mux : Mux  Inputs=2
  Product : Product
  Product1 : Product
  Product2 : Product
  Saturation1 : Saturate  UpperLimit=IM.Wr_rated*1.5  LowerLimit=-IM.Wr_rated*1.5
  Saturation2 : Saturate  UpperLimit=IM.Vs_rated  LowerLimit=-IM.Vs_rated
  Sin : Trigonometry
  Unit Delay : UnitDelay  SampleTime=-1  HasFrameUpgradeWarning=on
  Vdqss* : Outport
  wires:
  Wrpm*/1 -> Gain/1
  Gain/1 -> [Wrm_cmd]
  [Wrm_cmd] -> Gain1/1
  Gain1/1 -> [Wr_cmd]
  [Wr_cmd] -> If/1
  If Action Subsystem/1(Wr) -> Merge/1
  If Action Subsystem1/1(Wr) -> Merge/2
  If Action Subsystem2/1(Wr) -> Merge/3
  If/1 -> [acc]
  If/2 -> [dcc]
  If/3 -> [coast]
  [acc] -> If Action Subsystem/Action
  [dcc] -> If Action Subsystem1/Action
  [coast] -> If Action Subsystem2/Action
  [Wr_ref] -> If Action Subsystem/1(Wr*)
  [Wr_ref] -> If Action Subsystem1/1(Wr*)
  [Wr_ref] -> If Action Subsystem2/1(Wr*)
  IC/1 -> If/2
  [Wr_ref] -> IC/1
  [Wr_ref] -> Divide/1
  Constant/1 -> Divide/2
  Divide/1 -> Product/2
  Constant1/1 -> Product/1
  Product/1 -> Saturation2/1
  [Wr_ref] -> Saturation1/1
  Saturation1/1 -> [VF_Wr]
  [VF_Wr] -> Discrete-Time Integrator1/1
  Discrete-Time Integrator1/1 -> Bound PI/1(In)
  Bound PI/1(Out) -> [VF_Thetar]
  [VF_Thetar] -> Sin/1, Cos/1
  Cos/1 -> Product1/2
  Sin/1 -> Product2/2
  [VF_voltage] -> Product2/1, Product1/1
  Product1/1 -> [Vdss_Ref]
  Product2/1 -> [Vqss_Ref]
  Mux/1 -> Vdqss*/1
  [Vdss_Ref] -> Mux/1
  [Vqss_Ref] -> Mux/2
  Unit Delay/1 -> [Wr_ref]
  Merge/1 -> Unit Delay/1
  Saturation2/1 -> [VF_voltage]

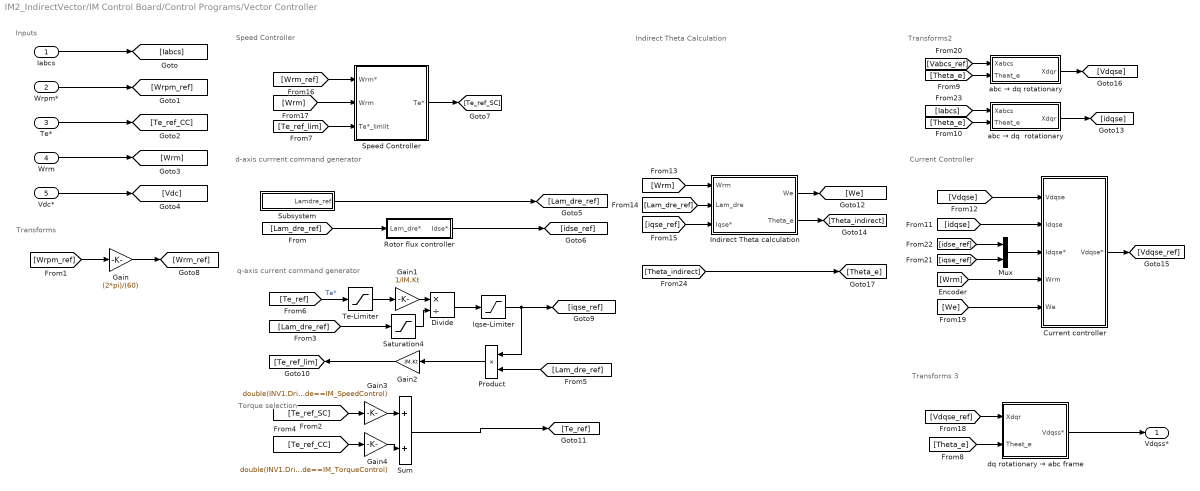
== system IM2_IndirectVector/IM Control Board/Control Programs/Vector Controller ==
  note: Current Controller
  note: Transforms2
  note: Transforms 3
  note: q-axis current command generator
  note: Torque selection
  note: Transforms
  note: d-axis currrent command generator
  note: Speed Controller
  note: Inputs
  note: Indirect Theta Calculation
  Iabcs : Inport
  Wrpm* : Inport  Port=2
  Te* : Inport  Port=3
  Wrm : Inport  Port=4
  Vdc* : Inport  Port=5
  "Current controller " : Subsystem
  Divide : Product  Inputs=*/
  Gain : Gain  Gain=(2*pi)/(60)
  Gain1 : Gain  Gain=1/IM.Kt
  Gain2 : Gain  Gain=IM.Kt
  Gain3 : Gain  Gain=double(INV1.DriveMode==IM_SpeedControl)
  Gain4 : Gain  Gain=double(INV1.DriveMode==IM_TorqueControl)
  Indirect Theta calculation : Subsystem
  Iqse-Limiter : Saturate  UpperLimit=IM.Iqse_rated  LowerLimit=-IM.Iqse_rated
  Mux : Mux  Inputs=2
  Product : Product
  Rotor flux controller : Subsystem
  Saturation4 : Saturate  UpperLimit=inf  LowerLimit=1e-04
  Speed Controller : Subsystem
  Subsystem : Subsystem
  Sum : Sum
  Te-Limiter : Saturate  UpperLimit=IM.Te_rated  LowerLimit=-IM.Te_rated
  abc → dq  rotationary : Subsystem
  abc → dq rotationary : Subsystem
  dq rotationary → abc frame : Subsystem
  Vdqss* : Outport
  wires:
  Iabcs/1 -> [Iabcs]
  Wrpm*/1 -> [Wrpm_ref]
  Te*/1 -> [Te_ref_CC]
  Wrm/1 -> [Wrm]
  Vdc*/1 -> [Vdc]
  Rotor flux controller/1(Idse*) -> [idse_ref]
  [Lam_dre_ref] -> Rotor flux controller/1(Lam_dre*)
  [Wrm_ref] -> Speed Controller/1(Wrm*)
  [Wrm] -> Speed Controller/2("Wrm ")
  Speed Controller/1(Te*) -> [Te_ref_SC]
  Gain/1 -> [Wrm_ref]
  [Wrpm_ref] -> Gain/1
  Product/1 -> Gain2/1
  Gain2/1 -> [Te_ref_lim]
  Divide/1 -> Iqse-Limiter/1
  Gain1/1 -> Divide/1
  Saturation4/1 -> Divide/2
  [Te_ref] -> Te-Limiter/1  "Te*"
  Iqse-Limiter/1 -> [iqse_ref], Product/1
  Te-Limiter/1 -> Gain1/1
  [Lam_dre_ref] -> Product/2
  [Lam_dre_ref] -> Saturation4/1
  Subsystem/1(Lamdre_ref) -> [Lam_dre_ref]
  [Te_ref_SC] -> Gain3/1
  [Te_ref_CC] -> Gain4/1
  Gain3/1 -> Sum/1
  Gain4/1 -> Sum/2
  Sum/1 -> [Te_ref]
  [Te_ref_lim] -> Speed Controller/3(Te*_limlit)
  [Iabcs] -> abc → dq  rotationary/1(Xabcs)
  abc → dq  rotationary/1(Xdqr) -> [idqse]
  [Vabcs_ref] -> abc → dq rotationary/1(Xabcs)
  [Wrm] -> "Current controller "/4(Wrm)
  [We] -> "Current controller "/5(We)
  [Theta_e] -> dq rotationary → abc frame/2("Theat_e ")
  Mux/1 -> "Current controller "/3(Idqse*)
  [idse_ref] -> Mux/1
  dq rotationary → abc frame/1(Vdqss*) -> Vdqss*/1
  [Theta_e] -> abc → dq  rotationary/2(Theat_e)
  "Current controller "/1(Vdqse*) -> [Vdqse_ref]
  [Theta_e] -> abc → dq rotationary/2(Theat_e)
  [iqse_ref] -> Mux/2
  abc → dq rotationary/1(Xdqr) -> [Vdqse]
  [Vdqse_ref] -> dq rotationary → abc frame/1(Xdqr)
  [idqse] -> "Current controller "/2(Idqse)
  [Vdqse] -> "Current controller "/1(Vdqse)
  [Lam_dre_ref] -> Indirect Theta calculation/2(Lam_dre)
  [iqse_ref] -> Indirect Theta calculation/3(Iqse*)
  [Wrm] -> Indirect Theta calculation/1(Wrm)
  Indirect Theta calculation/1(We) -> [We]
  Indirect Theta calculation/2(Theta_e) -> [Theta_indirect]
  [Theta_indirect] -> [Theta_e]

== system IM2_IndirectVector/IM Control Board/Control Programs/PWM/Vsn : Min//Max ==
  Vabcs* : Inport
  Add3 : Sum
  Gain1 : Gain  Gain=-0.5
  MinMax1 : MinMax  Function=max
  MinMax2 : MinMax
  Vsn* : Outport
  wires:
  Add3/1 -> Gain1/1
  MinMax2/1 -> Add3/2
  MinMax1/1 -> Add3/1
  [Vabcs_Ref] -> MinMax1/1, MinMax2/1
  Gain1/1 -> Vsn*/1
  Vabcs*/1 -> [Vabcs_Ref]

== system IM2_IndirectVector/IM Control Board/Control Programs/VF Control/Bound PI ==
  In : Inport
  Fcn1 : Fcn  Expr=1/(2*pi)*u+0.5
  Fcn2 : Fcn  Expr=u-floor(u)
  Fcn3 : Fcn  Expr=2*pi*(u-0.5)
  Out : Outport
  wires:
  Fcn1/1 -> Fcn2/1
  Fcn2/1 -> Fcn3/1
  In/1 -> Fcn1/1
  Fcn3/1 -> Out/1

== system IM2_IndirectVector/IM Control Board/Control Programs/VF Control/If Action Subsystem ==
  Wr* : Inport
  Action Port : ActionPort  ActionPortLabel=if(u1 > u2)
  Add : Sum  Inputs=|++
  Constant : Constant  Value=IM.acc_rate
  Gain : Gain  Gain=INV1.Tsw
  Wr : Outport
  wires:
  Wr*/1 -> Add/1
  Add/1 -> Wr/1
  Constant/1 -> Gain/1
  Gain/1 -> Add/2

== system IM2_IndirectVector/IM Control Board/Control Programs/VF Control/If Action Subsystem1 ==
  Wr* : Inport
  Action Port : ActionPort  ActionPortLabel=elseif(u1 < u2)
  Add : Sum  Inputs=|+-
  Constant : Constant  Value=IM.acc_rate
  Gain : Gain  Gain=INV1.Tsw
  Wr : Outport
  wires:
  Wr*/1 -> Add/1
  Constant/1 -> Gain/1
  Add/1 -> Wr/1
  Gain/1 -> Add/2

== system IM2_IndirectVector/IM Control Board/Control Programs/VF Control/If Action Subsystem2 ==
  Wr* : Inport
  Action Port : ActionPort  ActionPortLabel=else
  Wr : Outport
  wires:
  Wr*/1 -> Wr/1

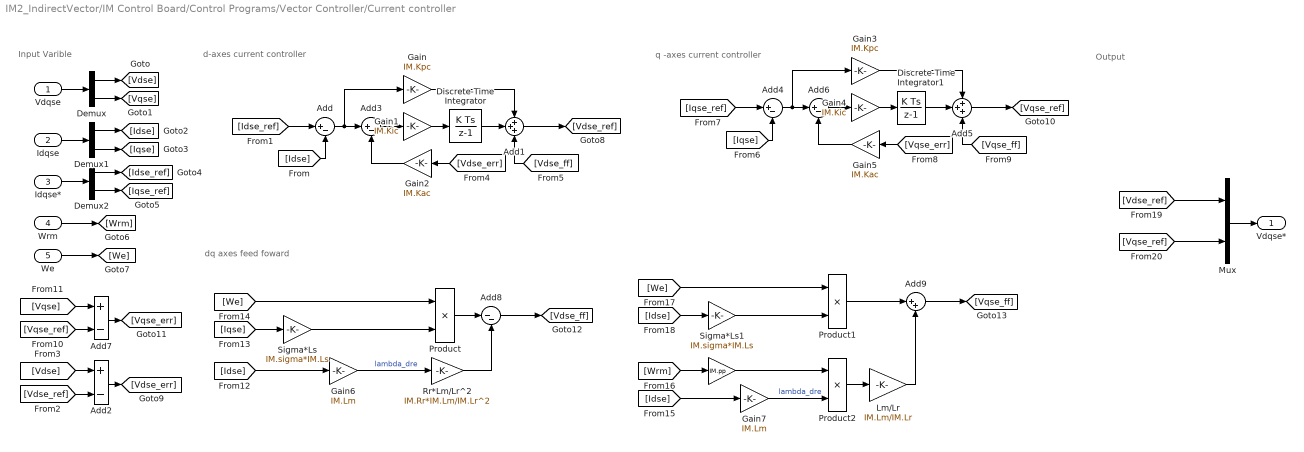
== system IM2_IndirectVector/IM Control Board/Control Programs/Vector Controller/Current controller  ==
  note: Output
  note: q -axes current controller
  note: d-axes current controller
  note: dq axes feed foward
  note: Input Varible
  Vdqse : Inport
  Idqse : Inport  Port=2
  Idqse* : Inport  Port=3
  Wrm : Inport  Port=4
  We : Inport  Port=5
  " " : Gain  Gain=IM.pp
  Add{,3..4,6} (4 alike) : Sum  Inputs=|+-
  Add1 : Sum  Inputs=+++
  Add2 : Sum  Inputs=+-
  Add5 : Sum  Inputs=+++
  Add7 : Sum  Inputs=+-
  Add8 : Sum  Inputs=|--
  Add9 : Sum  Inputs=|++
  Demux : Demux  Outputs=2
  Demux1 : Demux  Outputs=2
  Demux2 : Demux  Outputs=2
  Discrete-Time Integrator : DiscreteIntegrator  SampleTime=-1  ICPrevOutput=DiscIntNeverNeededParam  ICPrevScaledInput=DiscIntNeverNeededParam
  Discrete-Time Integrator1 : DiscreteIntegrator  SampleTime=-1  ICPrevOutput=DiscIntNeverNeededParam  ICPrevScaledInput=DiscIntNeverNeededParam
  Gain : Gain  Gain=IM.Kpc
  Gain1 : Gain  Gain=IM.Kic
  Gain2 : Gain  Gain=IM.Kac
  Gain3 : Gain  Gain=IM.Kpc
  Gain4 : Gain  Gain=IM.Kic
  Gain5 : Gain  Gain=IM.Kac
  Gain6 : Gain  Gain=IM.Lm
  Gain7 : Gain  Gain=IM.Lm
  Lm/Lr : Gain  Gain=IM.Lm/IM.Lr
  Mux : Mux  Inputs=2
  Product : Product
  Product1 : Product
  Product2 : Product
  "Rr*Lm/Lr^2 " : Gain  Gain=IM.Rr*IM.Lm/IM.Lr^2
  Sigma*Ls : Gain  Gain=IM.sigma*IM.Ls
  Sigma*Ls1 : Gain  Gain=IM.sigma*IM.Ls
  Vdqse* : Outport  VectorParamsAs1DForOutWhenUnconnected=off
  wires:
  Vdqse/1 -> Demux/1
  Demux/1 -> [Vdse]
  Demux/2 -> [Vqse]
  Demux1/1 -> [Idse]
  Idqse/1 -> Demux1/1
  Demux1/2 -> [Iqse]
  Demux2/1 -> [Idse_ref]
  Demux2/2 -> [Iqse_ref]
  Idqse*/1 -> Demux2/1
  Wrm/1 -> [Wrm]
  We/1 -> [We]
  [Idse] -> Add/2
  [Idse_ref] -> Add/1
  Add/1 -> Add3/1, Gain/1
  Gain1/1 -> Discrete-Time Integrator/1
  Discrete-Time Integrator/1 -> Add1/2
  Gain/1 -> Add1/1
  Add1/1 -> [Vdse_ref]
  [Vdse] -> Add2/1
  [Vdse_ref] -> Add2/2
  Add2/1 -> [Vdse_err]
  Add3/1 -> Gain1/1
  [Vdse_err] -> Gain2/1
  Gain2/1 -> Add3/2
  [Vdse_ff] -> Add1/3
  [Vqse_err] -> Gain5/1
  Gain5/1 -> Add6/2
  [Iqse] -> Add4/2
  Gain4/1 -> Discrete-Time Integrator1/1
  Add6/1 -> Gain4/1
  Add4/1 -> Add6/1, Gain3/1
  Add5/1 -> [Vqse_ref]
  Gain3/1 -> Add5/1
  [Iqse_ref] -> Add4/1
  Discrete-Time Integrator1/1 -> Add5/2
  [Vqse_ff] -> Add5/3
  [Vqse_ref] -> Add7/2
  Add7/1 -> [Vqse_err]
  [Vqse] -> Add7/1
  Add8/1 -> [Vdse_ff]
  "Rr*Lm/Lr^2 "/1 -> Add8/2
  [Idse] -> Gain6/1
  Gain6/1 -> "Rr*Lm/Lr^2 "/1  "lambda_dre"
  Product/1 -> Add8/1
  [Iqse] -> Sigma*Ls/1
  Sigma*Ls/1 -> Product/2
  [We] -> Product/1
  Product1/1 -> Add9/1
  Add9/1 -> [Vqse_ff]
  Lm/Lr/1 -> Add9/2
  Product2/1 -> Lm/Lr/1
  [Idse] -> Gain7/1
  Gain7/1 -> Product2/2  "lambda_dre"
  [Wrm] -> " "/1
  " "/1 -> Product2/1
  [We] -> Product1/1
  Sigma*Ls1/1 -> Product1/2
  [Idse] -> Sigma*Ls1/1
  Mux/1 -> Vdqse*/1
  [Vdse_ref] -> Mux/1
  [Vqse_ref] -> Mux/2

== system IM2_IndirectVector/IM Control Board/Control Programs/Vector Controller/Indirect Theta calculation ==
  Wrm : Inport
  Lam_dre : Inport  Port=2
  Iqse* : Inport  Port=3
  Add : Sum  Inputs=|++
  Divide : Product  Inputs=*/
  Gain : Gain  Gain=IM.pp
  Integrator : Subsystem
  Rr*Lm/Lr : Gain  Gain=IM.Lm/IM.Lr*IM.Rr
  Saturation4 : Saturate  UpperLimit=inf  LowerLimit=1e-04
  We : Outport  VectorParamsAs1DForOutWhenUnconnected=off
  Theta_e : Outport  Port=2  VectorParamsAs1DForOutWhenUnconnected=off
  wires:
  Iqse*/1 -> Rr*Lm/Lr/1
  Lam_dre/1 -> Saturation4/1
  Saturation4/1 -> Divide/2
  Rr*Lm/Lr/1 -> Divide/1
  Divide/1 -> Add/1  "Wsl"
  Wrm/1 -> Gain/1
  Gain/1 -> Add/2  "Wr"
  Add/1 -> Integrator/1(We), We/1
  Integrator/1(Theta_e) -> Theta_e/1

== system IM2_IndirectVector/IM Control Board/Control Programs/Vector Controller/Rotor flux controller ==
  Lam_dre* : Inport
  Gain : Gain  Gain=1/IM.Lm
  Idse* : Outport  VectorParamsAs1DForOutWhenUnconnected=off
  wires:
  Gain/1 -> Idse*/1
  Lam_dre*/1 -> Gain/1

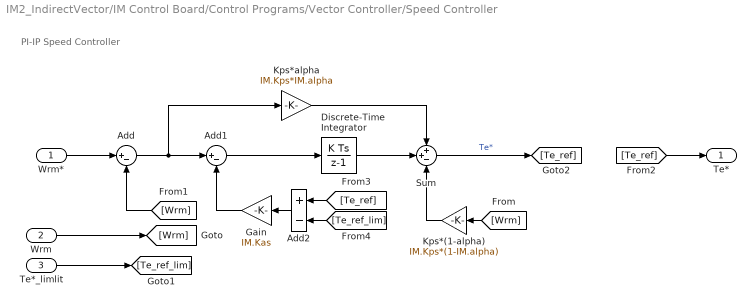
== system IM2_IndirectVector/IM Control Board/Control Programs/Vector Controller/Speed Controller ==
  note: PI-IP Speed Controller
  Wrm* : Inport
  "Wrm " : Inport  Port=2
  Te*_limlit : Inport  Port=3
  Add : Sum  Inputs=|+-
  Add1 : Sum  Inputs=|+-
  Add2 : Sum  Inputs=+-
  Discrete-Time Integrator : DiscreteIntegrator  SampleTime=-1  ICPrevOutput=DiscIntNeverNeededParam  ICPrevScaledInput=DiscIntNeverNeededParam
  Gain : Gain  Gain=IM.Kas
  Kps*(1-alpha) : Gain  Gain=IM.Kps*(1-IM.alpha)
  Kps*alpha : Gain  Gain=IM.Kps*IM.alpha
  Sum : Sum  Inputs=++-
  Te* : Outport  VectorParamsAs1DForOutWhenUnconnected=off
  wires:
  Wrm*/1 -> Add/1
  "Wrm "/1 -> [Wrm]
  Add/1 -> Kps*alpha/1, Add1/1
  Gain/1 -> Add1/2
  Add1/1 -> Discrete-Time Integrator/1
  Discrete-Time Integrator/1 -> Sum/2
  Kps*(1-alpha)/1 -> Sum/3
  Kps*alpha/1 -> Sum/1
  [Wrm] -> Add/2
  [Wrm] -> Kps*(1-alpha)/1
  Add2/1 -> Gain/1
  Sum/1 -> [Te_ref]  "Te*"
  [Te_ref] -> Add2/1
  [Te_ref_lim] -> Add2/2
  [Te_ref] -> Te*/1
  Te*_limlit/1 -> [Te_ref_lim]

== system IM2_IndirectVector/IM Control Board/Control Programs/Vector Controller/Subsystem ==
  Step1 : Step  Time=0  After=IM.Lam_dre_rated
  Lamdre_ref : Outport
  wires:
  Step1/1 -> Lamdre_ref/1

== system IM2_IndirectVector/IM Control Board/Control Programs/Vector Controller/abc → dq  rotationary ==
  Xabcs : Inport
  Theat_e : Inport  Port=2
  abc frame → dq staitionary : Subsystem
  dq stationary → rotationary : Subsystem
  Xdqr : Outport  VectorParamsAs1DForOutWhenUnconnected=off
  wires:
  Xabcs/1 -> abc frame → dq staitionary/1(Xabcs)
  abc frame → dq staitionary/1(Xdqs) -> dq stationary → rotationary/1(Xdqs)
  Theat_e/1 -> dq stationary → rotationary/2(Theta_e)
  dq stationary → rotationary/1(Xdqr) -> Xdqr/1

== system IM2_IndirectVector/IM Control Board/Control Programs/Vector Controller/abc → dq rotationary ==
  Xabcs : Inport
  Theat_e : Inport  Port=2
  abc frame → dq staitionary : Subsystem
  dq stationary → rotationary : Subsystem
  Xdqr : Outport  VectorParamsAs1DForOutWhenUnconnected=off
  wires:
  Xabcs/1 -> abc frame → dq staitionary/1(Xabcs)
  abc frame → dq staitionary/1(Xdqs) -> dq stationary → rotationary/1(Xdqs)
  Theat_e/1 -> dq stationary → rotationary/2(Theta_e)
  dq stationary → rotationary/1(Xdqr) -> Xdqr/1

== system IM2_IndirectVector/IM Control Board/Control Programs/Vector Controller/dq rotationary → abc frame ==
  Xdqr : Inport
  "Theat_e " : Inport  Port=2
  dq rotatinoary → dq stationary : Subsystem
  Vdqss* : Outport  VectorParamsAs1DForOutWhenUnconnected=off
  wires:
  "Theat_e "/1 -> dq rotatinoary → dq stationary/2(Theta_e)
  Xdqr/1 -> dq rotatinoary → dq stationary/1(Xdqr)
  dq rotatinoary → dq stationary/1(Xdqs) -> Vdqss*/1

== system IM2_IndirectVector/IM Control Board/Control Programs/Vector Controller/Indirect Theta calculation/Integrator ==
  We : Inport
  Discrete-Time Integrator : DiscreteIntegrator  SampleTime=-1  ICPrevOutput=DiscIntNeverNeededParam  ICPrevScaledInput=DiscIntNeverNeededParam
  bound pi : Subsystem
  Theta_e : Outport  VectorParamsAs1DForOutWhenUnconnected=off
  wires:
  We/1 -> Discrete-Time Integrator/1
  Discrete-Time Integrator/1 -> bound pi/1(theta)
  bound pi/1(bounded_theta) -> Theta_e/1

== system IM2_IndirectVector/IM Control Board/Control Programs/Vector Controller/abc → dq  rotationary/abc frame → dq staitionary ==
  Xabcs : Inport
  Add : Sum  Inputs=+--
  Add1 : Sum  Inputs=+-
  Demux : Demux  Outputs=3
  Gain : Gain  Gain=2
  Gain1 : Gain  Gain=1/3
  Gain2 : Gain  Gain=1/sqrt(3)
  Mux : Mux  Inputs=2
  Xdqs : Outport  VectorParamsAs1DForOutWhenUnconnected=off
  wires:
  Demux/1 -> Gain/1
  Gain/1 -> Add/1
  Demux/2 -> Add1/1, Add/2
  Demux/3 -> Add1/2, Add/3
  Add/1 -> Gain1/1
  Gain1/1 -> Mux/1
  Gain2/1 -> Mux/2
  Add1/1 -> Gain2/1
  Mux/1 -> Xdqs/1
  Xabcs/1 -> Demux/1

== system IM2_IndirectVector/IM Control Board/Control Programs/Vector Controller/abc → dq  rotationary/dq stationary → rotationary ==
  Xdqs : Inport
  Theta_e : Inport  Port=2
  Add : Sum  Inputs=++|
  Add1 : Sum  Inputs=|-+
  Cos : Trigonometry  Operator=cos
  Demux : Demux  Outputs=2
  Mux : Mux  Inputs=2
  Product{,1..3} (4 alike) : Product
  Sin : Trigonometry
  Xdqr : Outport  VectorParamsAs1DForOutWhenUnconnected=off
  wires:
  Xdqs/1 -> Demux/1
  Demux/1 -> Product2/1, Product/1  "Xds"
  Demux/2 -> Product3/1, Product1/1  "Xqs"
  Theta_e/1 -> Sin/1, Cos/1
  Cos/1 -> Product3/2, Product/2
  Product/1 -> Add/1
  Product1/1 -> Add/2
  Product2/1 -> Add1/1
  Product3/1 -> Add1/2
  Add1/1 -> Mux/2
  Add/1 -> Mux/1
  Sin/1 -> Product2/2, Product1/2
  Mux/1 -> Xdqr/1

== system IM2_IndirectVector/IM Control Board/Control Programs/Vector Controller/abc → dq rotationary/abc frame → dq staitionary ==
  Xabcs : Inport
  Add : Sum  Inputs=+--
  Add1 : Sum  Inputs=+-
  Demux : Demux  Outputs=3
  Gain : Gain  Gain=2
  Gain1 : Gain  Gain=1/3
  Gain2 : Gain  Gain=1/sqrt(3)
  Mux : Mux  Inputs=2
  Xdqs : Outport  VectorParamsAs1DForOutWhenUnconnected=off
  wires:
  Demux/1 -> Gain/1
  Gain/1 -> Add/1
  Demux/2 -> Add1/1, Add/2
  Demux/3 -> Add1/2, Add/3
  Add/1 -> Gain1/1
  Gain1/1 -> Mux/1
  Gain2/1 -> Mux/2
  Add1/1 -> Gain2/1
  Mux/1 -> Xdqs/1
  Xabcs/1 -> Demux/1

== system IM2_IndirectVector/IM Control Board/Control Programs/Vector Controller/abc → dq rotationary/dq stationary → rotationary ==
  Xdqs : Inport
  Theta_e : Inport  Port=2
  Add : Sum  Inputs=++|
  Add1 : Sum  Inputs=|-+
  Cos : Trigonometry  Operator=cos
  Demux : Demux  Outputs=2
  Mux : Mux  Inputs=2
  Product{,1..3} (4 alike) : Product
  Sin : Trigonometry
  Xdqr : Outport  VectorParamsAs1DForOutWhenUnconnected=off
  wires:
  Xdqs/1 -> Demux/1
  Demux/1 -> Product2/1, Product/1  "Xds"
  Demux/2 -> Product3/1, Product1/1  "Xqs"
  Theta_e/1 -> Sin/1, Cos/1
  Cos/1 -> Product3/2, Product/2
  Product/1 -> Add/1
  Product1/1 -> Add/2
  Product2/1 -> Add1/1
  Product3/1 -> Add1/2
  Add1/1 -> Mux/2
  Add/1 -> Mux/1
  Sin/1 -> Product2/2, Product1/2
  Mux/1 -> Xdqr/1

== system IM2_IndirectVector/IM Control Board/Control Programs/Vector Controller/dq rotationary → abc frame/dq rotatinoary → dq stationary ==
  Xdqr : Inport
  Theta_e : Inport  Port=2
  Demux : Demux  Outputs=2
  Divide{,1..3} (4 alike) : Product  Inputs=**
  Mux1 : Mux  Inputs=2
  Sum1 : Sum  Inputs=+-|
  Sum2 : Sum  Inputs=|++
  Trigonometric Function : Trigonometry  Operator=cos
  Trigonometric Function1 : Trigonometry
  Xdqs : Outport  VectorParamsAs1DForOutWhenUnconnected=off
  wires:
  Xdqr/1 -> Demux/1
  Mux1/1 -> Xdqs/1
  Divide3/1 -> Sum2/2
  Sum2/1 -> Mux1/2
  Divide2/1 -> Sum2/1
  Divide/1 -> Sum1/1
  Sum1/1 -> Mux1/1
  Divide1/1 -> Sum1/2
  Theta_e/1 -> Trigonometric Function/1, Trigonometric Function1/1
  Trigonometric Function/1 -> Divide3/2, Divide/2
  Demux/1 -> Divide2/1, Divide/1  "Xds"
  Demux/2 -> Divide3/1, Divide1/1  "Xqs"
  Trigonometric Function1/1 -> Divide2/2, Divide1/2

== system IM2_IndirectVector/IM Control Board/Control Programs/Vector Controller/Indirect Theta calculation/Integrator/bound pi ==
  theta : Inport
  Gain1 : Gain  Gain=2*pi
  Gain2 : Gain  Gain=1/(2*pi)
  Rounding Function : Rounding  Operator=round
  Subtract : Sum  Inputs=+-
  bounded_theta : Outport  VectorParamsAs1DForOutWhenUnconnected=off
  wires:
  Gain1/1 -> Subtract/2
  theta/1 -> Gain2/1, Subtract/1
  Rounding Function/1 -> Gain1/1
  Gain2/1 -> Rounding Function/1
  Subtract/1 -> bounded_theta/1
